simulink model "Blimp_Model"  (R2024b)
settings: Solver=ode4  StartTime=0.0  StopTime=10.0  FixedStep=0.01  RelTol=1e-3
settings Model: Creator=Alany  LastModifiedBy=Alany
settings SolverCC: ZeroCrossControl=DisableAll

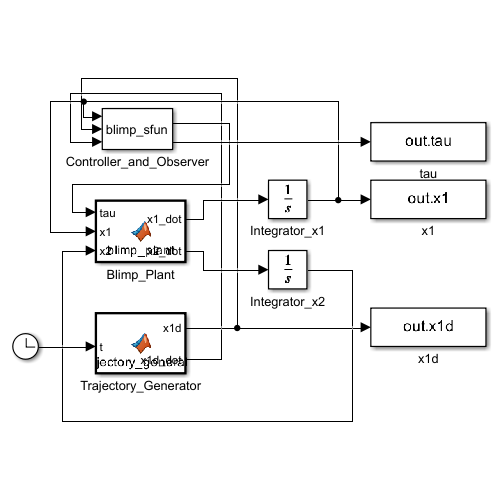
[thumbnail: Simulink's stored preview of the top-level diagram]
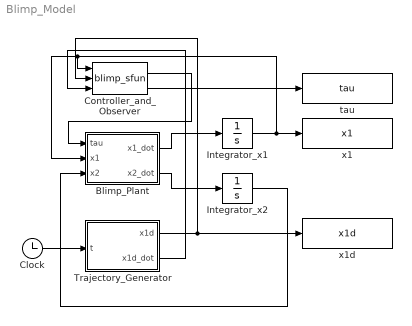
== system Blimp_Model ==
  Blimp_Plant : MATLAB Function  TreatAsAtomicUnit=on
  Clock : Clock
  Controller_and_Observer : M-S-Function  FunctionName=blimp_sfun  Parameters=W_in, W_d
  Integrator_x1 : Integrator  InitialCondition=[1.3; -0.1; -0.06; -0.03]
  Integrator_x2 : Integrator  InitialCondition=[0; 0; 0; 0]
  Trajectory_Generator : MATLAB Function  TreatAsAtomicUnit=on
  tau : ToWorkspace  VariableName=tau  SampleTime=-1
  x1 : ToWorkspace  VariableName=x1  SampleTime=-1
  x1d : ToWorkspace  VariableName=x1d  SampleTime=-1
  wires:
  Clock/1 -> Trajectory_Generator/1(t)
  Trajectory_Generator/1(x1d) -> x1d/1, Controller_and_Observer/2
  Trajectory_Generator/2(x1d_dot) -> Controller_and_Observer/3
  Controller_and_Observer/1 -> Blimp_Plant/1(tau)
  Blimp_Plant/1(x1_dot) -> Integrator_x1/1
  Blimp_Plant/2(x2_dot) -> Integrator_x2/1
  Integrator_x2/1 -> Blimp_Plant/3(x2)
  Integrator_x1/1 -> x1/1, Controller_and_Observer/1, Blimp_Plant/2(x1)
  Controller_and_Observer/2 -> tau/1

== matlab function Blimp_Model/Blimp_Plant ==
  data: tau input; x1_dot output; x1 input; x2 input; x2_dot output
function [x1_dot, x2_dot] = blimp_plant(tau, x1, x2)
    % 提取状态
    psi = x1(4);
    vx = x2(1); vy = x2(2); vz = x2(3); wz = x2(4);
    
    % 旋转矩阵
    J = [cos(psi), -sin(psi), 0, 0; 
         sin(psi), cos(psi), 0, 0; 
         0, 0, 1, 0; 
         0, 0, 0, 1];
    
    % 物理参数
    m_R = 0.884; m_Ax = 0.585; m_Ay = 0.585; m_Az = 0.607;
    I_RBz = 0.039; I_Az = 0.012; x_g = 0.05;
    
    % 惯性矩阵 M
    M = diag([m_R+m_Ax, m_R+m_Ay, m_R+m_Az, I_RBz+I_Az]);
    M(2,4) = m_R*x_g; M(4,2) = m_R*x_g;
    
    % 科里奥利矩阵 C
    C = zeros(4,4);
    C(1,4) = -(m_R+m_Ay)*vy - m_R*x_g*wz; 
    C(4,1) = -C(1,4);
    C(2,4) = (m_R+m_Ax)*vx; 
    C(4,2) = -C(2,4);
    
    % 阻尼矩阵 D 和重力/浮力 g
    D = diag([0.031, 0.031, 0.025, 0.001]);
    g_vec = [0; 0; 0; 0]; % fG - fB = 0
    
    % 动力学方程：求加速度和速度
    x2_dot = M \ (tau - C*x2 - D*x2 - g_vec);
    x1_dot = J * x2;
end

== matlab function Blimp_Model/Trajectory_Generator ==
  data: t input; x1d output; x1d_dot output
function [x1d, x1d_dot] = trajectory_generator(t)
    % 论文 Exp1-Test1 圆形轨迹
    % x1d = [x; y; z; psi]
    x = 1.2 * cos(0.05*t);
    y = 1.2 * sin(0.05*t);
    z = 0.6 + 0.03 * log(cosh(t-5) / cosh(t-25));
    psi = -0.03; % 假设初始偏航角保持不变
    x1d = [x; y; z; psi];
    
    % 期望轨迹的导数 (速度)
    dx = -1.2 * 0.05 * sin(0.05*t);
    dy = 1.2 * 0.05 * cos(0.05*t);
    dz = 0.03 * (tanh(t-5) - tanh(t-25));
    dpsi = 0;
    x1d_dot = [dx; dy; dz; dpsi];
end
